simulink model "hex"  (R2014b)
settings: Solver=ode45  StartTime=0.0  StopTime=10.0  RelTol=1e-3
settings Model: Creator=dell  LastModifiedBy=dell

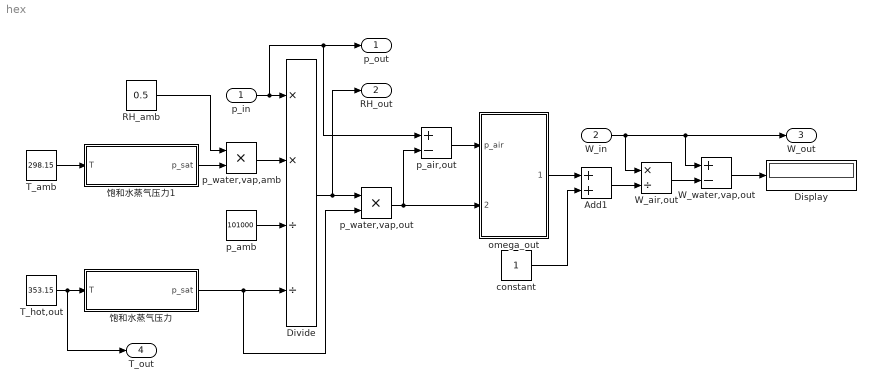
== system hex ==
  p_in : Inport
  W_in : Inport  Port=2
  Add1 : Sum
  Display : Display
  Divide : Product  Inputs=**//
  RH_amb : Constant  Value=0.5
  T_amb : Constant  Value=298.15
  T_hot,out : Constant  Value=353.15
  W_air,out : Product  Inputs=*/
  W_water,vap,out : Sum  Inputs=+-
  "constant " : Constant
  omega_out : Subsystem
  p_air,out : Sum  Inputs=+-
  p_amb : Constant  Value=101000
  p_water,vap,amb : Product
  p_water,vap,out : Product
  饱和水蒸气压力 : Subsystem
  饱和水蒸气压力1 : Subsystem
  p_out : Outport
  RH_out : Outport  Port=2
  W_out : Outport  Port=3
  T_out : Outport  Port=4
  wires:
  T_hot,out/1 -> T_out/1, 饱和水蒸气压力/1(T)
  T_amb/1 -> 饱和水蒸气压力1/1(T)
  饱和水蒸气压力1/1(p_sat) -> p_water,vap,amb/2
  RH_amb/1 -> p_water,vap,amb/1
  p_in/1 -> Divide/1, p_out/1, p_air,out/1
  p_water,vap,amb/1 -> Divide/2
  p_amb/1 -> Divide/3
  Divide/1 -> RH_out/1, p_water,vap,out/1
  饱和水蒸气压力/1(p_sat) -> p_water,vap,out/2, Divide/4
  p_water,vap,out/1 -> omega_out/2(p_water), p_air,out/2
  p_air,out/1 -> omega_out/1(p_air)
  omega_out/1(omega) -> Add1/1
  "constant "/1 -> Add1/2
  Add1/1 -> W_air,out/2
  W_in/1 -> W_out/1, W_water,vap,out/1, W_air,out/1
  W_air,out/1 -> W_water,vap,out/2
  W_water,vap,out/1 -> Display/1

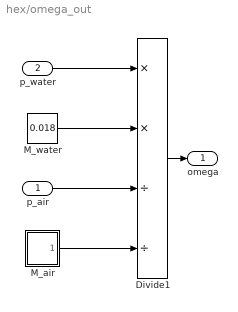
== system hex/omega_out ==
  p_air : Inport
  p_water : Inport  Port=2
  Divide1 : Product  Inputs=**//
  M_air : Subsystem
  M_water : Constant  Value=0.018
  omega : Outport
  wires:
  M_water/1 -> Divide1/2
  p_air/1 -> Divide1/3
  M_air/1(M_air) -> Divide1/4
  p_water/1 -> Divide1/1
  Divide1/1 -> omega/1

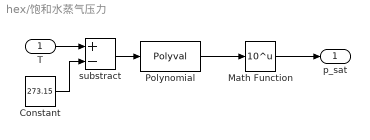
== system hex/饱和水蒸气压力 ==
  T : Inport
  Constant : Constant  Value=273.15
  Math Function : Math  Operator=10^u  SaturateOnIntegerOverflow=on
  Polynomial : Polyval  Coefs=[1.4454e-7,-9.1837e-5,0.2953,-2.1794]
  substract : Sum  Inputs=+-
  p_sat : Outport
  wires:
  Polynomial/1 -> Math Function/1
  T/1 -> substract/1
  Math Function/1 -> p_sat/1
  substract/1 -> Polynomial/1
  Constant/1 -> substract/2

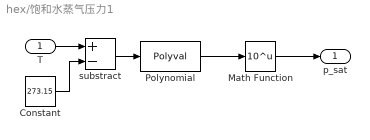
== system hex/饱和水蒸气压力1 ==
  T : Inport
  Constant : Constant  Value=273.15
  Math Function : Math  Operator=10^u  SaturateOnIntegerOverflow=on
  Polynomial : Polyval  Coefs=[1.4454e-7,-9.1837e-5,0.2953,-2.1794]
  substract : Sum  Inputs=+-
  p_sat : Outport
  wires:
  Polynomial/1 -> Math Function/1
  T/1 -> substract/1
  Math Function/1 -> p_sat/1
  substract/1 -> Polynomial/1
  Constant/1 -> substract/2

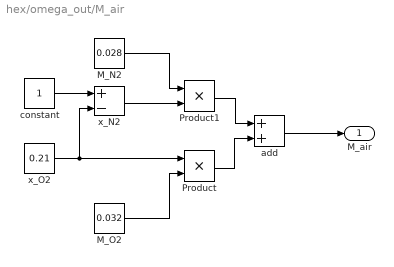
== system hex/omega_out/M_air ==
  M_N2 : Constant  Value=0.028
  M_O2 : Constant  Value=0.032
  Product : Product
  Product1 : Product
  add : Sum
  constant : Constant
  x_N2 : Sum  Inputs=+-
  x_O2 : Constant  Value=0.21
  M_air : Outport
  wires:
  constant/1 -> x_N2/1
  x_O2/1 -> Product/1, x_N2/2
  M_O2/1 -> Product/2
  M_N2/1 -> Product1/1
  x_N2/1 -> Product1/2
  Product/1 -> add/2
  Product1/1 -> add/1
  add/1 -> M_air/1
